simulink model "mdl4"  (Simulink 8.3)
settings: Solver=FixedStepDiscrete  SolverMode=SingleTasking  StartTime=TIME(1)  StopTime=TIME(end)  FixedStep=SIMSTEP  RelTol=1e-3
values from neighbouring files (symbols this model uses):
  Parameter113 = 123    [scr_simdata_all.mat]
  Parameter131 = 3    [scr_simdata_all.mat]
  Parameter132 = 100    [scr_simdata_all.mat]
  Parameter144 = 3    [scr_simdata_all.mat]
  Parameter51 = 0    [scr_simdata_all.mat]
  Parameter52 = 1    [scr_simdata_all.mat]
  Parameter53 = 2    [scr_simdata_all.mat]
  Parameter54 = 255    [scr_simdata_all.mat]
  Parameter69 = 27    [scr_simdata_all.mat]
  Parameter91 = 75    [scr_simdata_all.mat]
  SIMSTEP = 0.0001024    [scr_simdata_all.mat]
(part 2 of 4)

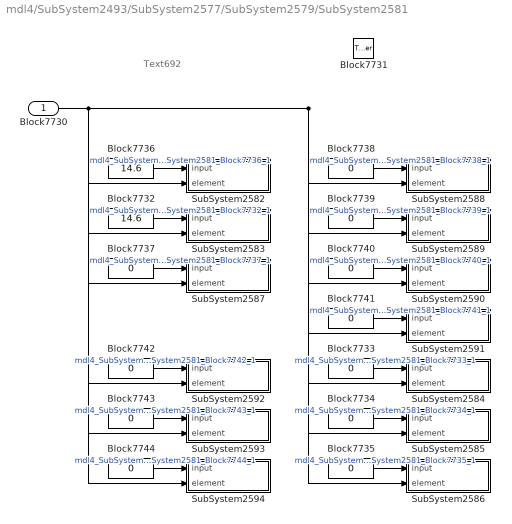
== system mdl4/SubSystem2493/SubSystem2577/SubSystem2579/SubSystem2581 ==
  note: Text692
  Block7730 : Inport
  Block7731 : TriggerPort  TriggerType=function-call
  Block7732 : Constant  Value=14.6  OutDataTypeStr=double  SampleTime=-1
  Block{7733..7735,7737..7744} (11 alike) : Constant  Value=0  OutDataTypeStr=double  SampleTime=-1
  Block7736 : Constant  Value=14.6  OutDataTypeStr=double  SampleTime=-1
  SubSystem2582 : Subsystem  TreatAsAtomicUnit=on  mask(***ATC.DSWVEC***){bd_version=1.01.A, r0=DSM258, r1=-1, r2=, r3=, r4=, r5=, r6=, r7=, r8=, r9=, c0=, c1=, c2=, c3=, c4=, c5=, c6=, c7=, c8=, c9=}
      mask prompts: bd_version "Version"
      mask help: これはAutoCからのブロックです．編集禁止．
      settings: OpenFcn=warndlg('変更禁止!');
      mask Help: web(ui_blockhelpmng(gcb));
      mask Display: disp('ATC.DSRVEC')
  SubSystem2583 : Subsystem  TreatAsAtomicUnit=on  mask(***ATC.DSWVEC***){bd_version=1.01.A, r0=DSM275, r1=-1, r2=, r3=, r4=, r5=, r6=, r7=, r8=, r9=, c0=, c1=, c2=, c3=, c4=, c5=, c6=, c7=, c8=, c9=}
      mask prompts: bd_version "Version"
      mask help: これはAutoCからのブロックです．編集禁止．
      settings: OpenFcn=warndlg('変更禁止!');
      mask Help: web(ui_blockhelpmng(gcb));
      mask Display: disp('ATC.DSRVEC')
  SubSystem2584 : Subsystem  TreatAsAtomicUnit=on  mask(***ATC.DSWVEC***){bd_version=1.01.A, r0=DSM295, r1=-1, r2=, r3=, r4=, r5=, r6=, r7=, r8=, r9=, c0=, c1=, c2=, c3=, c4=, c5=, c6=, c7=, c8=, c9=}
      mask prompts: bd_version "Version"
      mask help: これはAutoCからのブロックです．編集禁止．
      settings: OpenFcn=warndlg('変更禁止!');
      mask Help: web(ui_blockhelpmng(gcb));
      mask Display: disp('ATC.DSRVEC')
  SubSystem2585 : Subsystem  TreatAsAtomicUnit=on  mask(***ATC.DSWVEC***){bd_version=1.01.A, r0=DSM280, r1=-1, r2=, r3=, r4=, r5=, r6=, r7=, r8=, r9=, c0=, c1=, c2=, c3=, c4=, c5=, c6=, c7=, c8=, c9=}
      mask prompts: bd_version "Version"
      mask help: これはAutoCからのブロックです．編集禁止．
      settings: OpenFcn=warndlg('変更禁止!');
      mask Help: web(ui_blockhelpmng(gcb));
      mask Display: disp('ATC.DSRVEC')
  SubSystem2586 : Subsystem  TreatAsAtomicUnit=on  mask(***ATC.DSWVEC***){bd_version=1.01.A, r0=DSM282, r1=-1, r2=, r3=, r4=, r5=, r6=, r7=, r8=, r9=, c0=, c1=, c2=, c3=, c4=, c5=, c6=, c7=, c8=, c9=}
      mask prompts: bd_version "Version"
      mask help: これはAutoCからのブロックです．編集禁止．
      settings: OpenFcn=warndlg('変更禁止!');
      mask Help: web(ui_blockhelpmng(gcb));
      mask Display: disp('ATC.DSRVEC')
  SubSystem2587 : Subsystem  TreatAsAtomicUnit=on  mask(***ATC.DSWVEC***){bd_version=1.01.A, r0=DSM274, r1=-1, r2=, r3=, r4=, r5=, r6=, r7=, r8=, r9=, c0=, c1=, c2=, c3=, c4=, c5=, c6=, c7=, c8=, c9=}
      mask prompts: bd_version "Version"
      mask help: これはAutoCからのブロックです．編集禁止．
      settings: OpenFcn=warndlg('変更禁止!');
      mask Help: web(ui_blockhelpmng(gcb));
      mask Display: disp('ATC.DSRVEC')
  SubSystem2588 : Subsystem  TreatAsAtomicUnit=on  mask(***ATC.DSWVEC***){bd_version=1.01.A, r0=DSM302, r1=-1, r2=, r3=, r4=, r5=, r6=, r7=, r8=, r9=, c0=, c1=, c2=, c3=, c4=, c5=, c6=, c7=, c8=, c9=}
      mask prompts: bd_version "Version"
      mask help: これはAutoCからのブロックです．編集禁止．
      settings: OpenFcn=warndlg('変更禁止!');
      mask Help: web(ui_blockhelpmng(gcb));
      mask Display: disp('ATC.DSRVEC')
  SubSystem2589 : Subsystem  TreatAsAtomicUnit=on  mask(***ATC.DSWVEC***){bd_version=1.01.A, r0=DSM303, r1=-1, r2=, r3=, r4=, r5=, r6=, r7=, r8=, r9=, c0=, c1=, c2=, c3=, c4=, c5=, c6=, c7=, c8=, c9=}
      mask prompts: bd_version "Version"
      mask help: これはAutoCからのブロックです．編集禁止．
      settings: OpenFcn=warndlg('変更禁止!');
      mask Help: web(ui_blockhelpmng(gcb));
      mask Display: disp('ATC.DSRVEC')
  SubSystem2590 : Subsystem  TreatAsAtomicUnit=on  mask(***ATC.DSWVEC***){bd_version=1.01.A, r0=DSM300, r1=-1, r2=, r3=, r4=, r5=, r6=, r7=, r8=, r9=, c0=, c1=, c2=, c3=, c4=, c5=, c6=, c7=, c8=, c9=}
      mask prompts: bd_version "Version"
      mask help: これはAutoCからのブロックです．編集禁止．
      settings: OpenFcn=warndlg('変更禁止!');
      mask Help: web(ui_blockhelpmng(gcb));
      mask Display: disp('ATC.DSRVEC')
  SubSystem2591 : Subsystem  TreatAsAtomicUnit=on  mask(***ATC.DSWVEC***){bd_version=1.01.A, r0=DSM301, r1=-1, r2=, r3=, r4=, r5=, r6=, r7=, r8=, r9=, c0=, c1=, c2=, c3=, c4=, c5=, c6=, c7=, c8=, c9=}
      mask prompts: bd_version "Version"
      mask help: これはAutoCからのブロックです．編集禁止．
      settings: OpenFcn=warndlg('変更禁止!');
      mask Help: web(ui_blockhelpmng(gcb));
      mask Display: disp('ATC.DSRVEC')
  SubSystem2592 : Subsystem  TreatAsAtomicUnit=on  mask(***ATC.DSWVEC***){bd_version=1.01.A, r0=DSM293, r1=-1, r2=, r3=, r4=, r5=, r6=, r7=, r8=, r9=, c0=, c1=, c2=, c3=, c4=, c5=, c6=, c7=, c8=, c9=}
      mask prompts: bd_version "Version"
      mask help: これはAutoCからのブロックです．編集禁止．
      settings: OpenFcn=warndlg('変更禁止!');
      mask Help: web(ui_blockhelpmng(gcb));
      mask Display: disp('ATC.DSRVEC')
  SubSystem2593 : Subsystem  TreatAsAtomicUnit=on  mask(***ATC.DSWVEC***){bd_version=1.01.A, r0=DSM279, r1=-1, r2=, r3=, r4=, r5=, r6=, r7=, r8=, r9=, c0=, c1=, c2=, c3=, c4=, c5=, c6=, c7=, c8=, c9=}
      mask prompts: bd_version "Version"
      mask help: これはAutoCからのブロックです．編集禁止．
      settings: OpenFcn=warndlg('変更禁止!');
      mask Help: web(ui_blockhelpmng(gcb));
      mask Display: disp('ATC.DSRVEC')
  SubSystem2594 : Subsystem  TreatAsAtomicUnit=on  mask(***ATC.DSWVEC***){bd_version=1.01.A, r0=DSM281, r1=-1, r2=, r3=, r4=, r5=, r6=, r7=, r8=, r9=, c0=, c1=, c2=, c3=, c4=, c5=, c6=, c7=, c8=, c9=}
      mask prompts: bd_version "Version"
      mask help: これはAutoCからのブロックです．編集禁止．
      settings: OpenFcn=warndlg('変更禁止!');
      mask Help: web(ui_blockhelpmng(gcb));
      mask Display: disp('ATC.DSRVEC')
  wires:
  Block7736/1 -> SubSystem2582/1(input)  "mdl4_SubSystem2493_SubSystem2577_SubSystem2579_SubSystem2581_Block7736_1"
  Block7730/1 -> SubSystem2582/2(element), SubSystem2587/2(element), SubSystem2583/2(element), SubSystem2592/2(element), SubSystem2593/2(element), SubSystem2594/2(element), SubSystem2588/2(element), SubSystem2589/2(element), SubSystem2590/2(element), SubSystem2591/2(element), SubSystem2584/2(element), SubSystem2585/2(element), SubSystem2586/2(element)
  Block7732/1 -> SubSystem2583/1(input)  "mdl4_SubSystem2493_SubSystem2577_SubSystem2579_SubSystem2581_Block7732_1"
  Block7737/1 -> SubSystem2587/1(input)  "mdl4_SubSystem2493_SubSystem2577_SubSystem2579_SubSystem2581_Block7737_1"
  Block7738/1 -> SubSystem2588/1(input)  "mdl4_SubSystem2493_SubSystem2577_SubSystem2579_SubSystem2581_Block7738_1"
  Block7739/1 -> SubSystem2589/1(input)  "mdl4_SubSystem2493_SubSystem2577_SubSystem2579_SubSystem2581_Block7739_1"
  Block7740/1 -> SubSystem2590/1(input)  "mdl4_SubSystem2493_SubSystem2577_SubSystem2579_SubSystem2581_Block7740_1"
  Block7741/1 -> SubSystem2591/1(input)  "mdl4_SubSystem2493_SubSystem2577_SubSystem2579_SubSystem2581_Block7741_1"
  Block7742/1 -> SubSystem2592/1(input)  "mdl4_SubSystem2493_SubSystem2577_SubSystem2579_SubSystem2581_Block7742_1"
  Block7743/1 -> SubSystem2593/1(input)  "mdl4_SubSystem2493_SubSystem2577_SubSystem2579_SubSystem2581_Block7743_1"
  Block7744/1 -> SubSystem2594/1(input)  "mdl4_SubSystem2493_SubSystem2577_SubSystem2579_SubSystem2581_Block7744_1"
  Block7733/1 -> SubSystem2584/1(input)  "mdl4_SubSystem2493_SubSystem2577_SubSystem2579_SubSystem2581_Block7733_1"
  Block7734/1 -> SubSystem2585/1(input)  "mdl4_SubSystem2493_SubSystem2577_SubSystem2579_SubSystem2581_Block7734_1"
  Block7735/1 -> SubSystem2586/1(input)  "mdl4_SubSystem2493_SubSystem2577_SubSystem2579_SubSystem2581_Block7735_1"

== system mdl4/SubSystem2493/SubSystem2494/SubSystem2500/SubSystem2504/SubSystem2505 ==
  note: ***編集禁止***
  input : Inport
  element : Inport  Port=2
  Assignment : Assignment  IndexOptions=Index vector (port)  OutputSizes=[1 1]
  Inside_DSR : DataStoreRead  DataStoreName=DSM274
  Inside_DSW : DataStoreWrite  DataStoreName=DSM274
  wires:
  Assignment/1 -> Inside_DSW/1  "mdl4_SubSystem2493_SubSystem2494_SubSystem2500_SubSystem2504_SubSystem2505_Assignment_1"
  Inside_DSR/1 -> Assignment/1  "mdl4_SubSystem2493_SubSystem2494_SubSystem2500_SubSystem2504_SubSystem2505_Inside_DSR_1"
  input/1 -> Assignment/2
  element/1 -> Assignment/3

== system mdl4/SubSystem2493/SubSystem2494/SubSystem2500/SubSystem2504/SubSystem2506 ==
  note: ***編集禁止***
  In1 : Inport
  In2 : Inport  Port=2
  RO1 : RelationalOperator  Operator===  InputSameDT=on
  single1 : DataTypeConversion  OutDataTypeStr=single  SaturateOnIntegerOverflow=on  RndMeth=Zero
  single2 : DataTypeConversion  OutDataTypeStr=single  SaturateOnIntegerOverflow=on  RndMeth=Zero
  Out1 : Outport
  wires:
  single2/1 -> RO1/2  "mdl4_SubSystem2493_SubSystem2494_SubSystem2500_SubSystem2504_SubSystem2506_single2_1"
  single1/1 -> RO1/1  "mdl4_SubSystem2493_SubSystem2494_SubSystem2500_SubSystem2504_SubSystem2506_single1_1"
  In1/1 -> single1/1
  In2/1 -> single2/1
  RO1/1 -> Out1/1  "mdl4_SubSystem2493_SubSystem2494_SubSystem2500_SubSystem2504_SubSystem2506_RO1_1"

== system mdl4/SubSystem2493/SubSystem2494/SubSystem2500/SubSystem2504/SubSystem2507 ==
  note: Text615
  note: Text614
  note: Text613
  note: Text612
  Block7508 : Inport
  Block7509 : Constant  OutDataTypeStr=double  SampleTime=-1
  Block7510 : DataStoreRead  DataStoreName=DSM299
  Block7511 : DataStoreRead  DataStoreName=DSM297
  Block7512 : DataStoreRead  DataStoreName=DSM285
  Block7513 : DataStoreRead  DataStoreName=DSM283
  Block7514 : Demux  Outputs=2
  Block7517 : Sum  Inputs=+-|  OutDataTypeStr=double  RndMeth=Zero  SaturateOnIntegerOverflow=on  InputSameDT=on
  Block7518 : Switch  Threshold=0.5  RndMeth=Zero  SaturateOnIntegerOverflow=on  InputSameDT=on
  SubSystem2508 : Subsystem
  Block7519 : Outport
  Block7520 : Outport  Port=2
  Block7521 : Outport  Port=3
  Block7522 : Outport  Port=4
  wires:
  Block7510/1 -> SubSystem2508/1(In1)  "mdl4_SubSystem2493_SubSystem2494_SubSystem2500_SubSystem2504_SubSystem2507_Block7510_1"
  Block7509/1 -> SubSystem2508/2(In2)  "mdl4_SubSystem2493_SubSystem2494_SubSystem2500_SubSystem2504_SubSystem2507_Block7509_1"
  SubSystem2508/1(Out1) -> Block7518/2
  Block7508/1 -> Block7517/2
  Block7511/1 -> Block7517/1  "mdl4_SubSystem2493_SubSystem2494_SubSystem2500_SubSystem2504_SubSystem2507_Block7511_1"
  Block7517/1 -> Block7514/1  "mdl4_SubSystem2493_SubSystem2494_SubSystem2500_SubSystem2504_SubSystem2507_Block7517_1"
  Block7518/1 -> Block7519/1  "mdl4_SubSystem2493_SubSystem2494_SubSystem2500_SubSystem2504_SubSystem2507_Block7518_1"
  Block7514/1 -> Block7518/3, Block7520/1  "SigLabel273"
  Block7514/2 -> [TagName60]  "SigLabel270"
  [TagName60] -> Block7518/1  "SigLabel269"
  Block7512/1 -> Block7521/1  "mdl4_SubSystem2493_SubSystem2494_SubSystem2500_SubSystem2504_SubSystem2507_Block7512_1"
  Block7513/1 -> Block7522/1  "mdl4_SubSystem2493_SubSystem2494_SubSystem2500_SubSystem2504_SubSystem2507_Block7513_1"

== system mdl4/SubSystem2493/SubSystem2494/SubSystem2500/SubSystem2504/SubSystem2509 ==
  note: Text619
  note: Text618
  note: Text617
  note: Text616
  Block7523 : Inport
  Block7524 : Constant  OutDataTypeStr=double  SampleTime=-1
  Block7525 : DataStoreRead  DataStoreName=DSM299
  Block7526 : DataStoreRead  DataStoreName=DSM298
  Block7527 : DataStoreRead  DataStoreName=DSM286
  Block7528 : DataStoreRead  DataStoreName=DSM284
  Block7529 : Demux  Outputs=2
  Block7530 : Sum  Inputs=+-|  OutDataTypeStr=double  RndMeth=Zero  SaturateOnIntegerOverflow=on  InputSameDT=on
  Block7531 : Switch  Threshold=0.5  RndMeth=Zero  SaturateOnIntegerOverflow=on  InputSameDT=on
  SubSystem2510 : Subsystem
  Block7532 : Outport
  Block7533 : Outport  Port=2
  Block7534 : Outport  Port=3
  Block7535 : Outport  Port=4
  wires:
  Block7528/1 -> Block7535/1  "mdl4_SubSystem2493_SubSystem2494_SubSystem2500_SubSystem2504_SubSystem2509_Block7528_1"
  Block7527/1 -> Block7534/1  "mdl4_SubSystem2493_SubSystem2494_SubSystem2500_SubSystem2504_SubSystem2509_Block7527_1"
  Block7529/1 -> Block7533/1, Block7531/1  "SigLabel277"
  Block7531/1 -> Block7532/1  "mdl4_SubSystem2493_SubSystem2494_SubSystem2500_SubSystem2504_SubSystem2509_Block7531_1"
  Block7530/1 -> Block7529/1  "mdl4_SubSystem2493_SubSystem2494_SubSystem2500_SubSystem2504_SubSystem2509_Block7530_1"
  Block7526/1 -> Block7530/1  "mdl4_SubSystem2493_SubSystem2494_SubSystem2500_SubSystem2504_SubSystem2509_Block7526_1"
  Block7523/1 -> Block7530/2
  SubSystem2510/1(Out1) -> Block7531/2
  Block7524/1 -> SubSystem2510/2(In2)  "mdl4_SubSystem2493_SubSystem2494_SubSystem2500_SubSystem2504_SubSystem2509_Block7524_1"
  Block7525/1 -> SubSystem2510/1(In1)  "mdl4_SubSystem2493_SubSystem2494_SubSystem2500_SubSystem2504_SubSystem2509_Block7525_1"
  Block7529/2 -> Block7531/3  "SigLabel274"

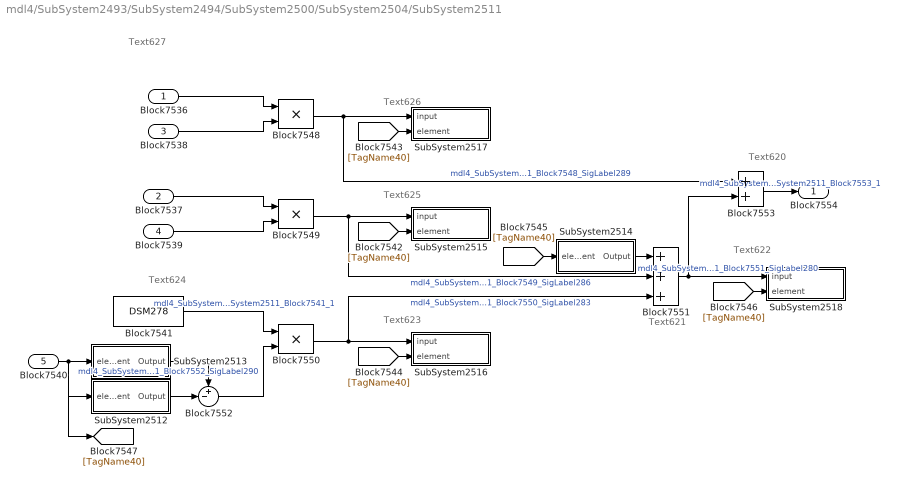
== system mdl4/SubSystem2493/SubSystem2494/SubSystem2500/SubSystem2504/SubSystem2511 ==
  note: Text627
  note: Text626
  note: Text625
  note: Text624
  note: Text623
  note: Text622
  note: Text621
  note: Text620
  Block7536 : Inport
  Block7537 : Inport  Port=2
  Block7538 : Inport  Port=3
  Block7539 : Inport  Port=4
  Block7540 : Inport  Port=5
  Block7541 : DataStoreRead  DataStoreName=DSM278
  Block7548 : Product  OutDataTypeStr=double  SaturateOnIntegerOverflow=on  RndMeth=Zero  InputSameDT=on
  Block7549 : Product  OutDataTypeStr=double  SaturateOnIntegerOverflow=on  RndMeth=Zero  InputSameDT=on
  Block7550 : Product  OutDataTypeStr=double  SaturateOnIntegerOverflow=on  RndMeth=Zero  InputSameDT=on
  Block7551 : Sum  Inputs=3  OutDataTypeStr=double  RndMeth=Zero  SaturateOnIntegerOverflow=on  InputSameDT=on
  Block7552 : Sum  Inputs=+-|  OutDataTypeStr=double  RndMeth=Zero  SaturateOnIntegerOverflow=on  InputSameDT=on
  Block7553 : Sum  Inputs=2  OutDataTypeStr=double  RndMeth=Zero  SaturateOnIntegerOverflow=on  InputSameDT=on
  SubSystem2512 : Subsystem  TreatAsAtomicUnit=on  mask(***ATC.DSRVEC***){bd_version=1.01.A, r0=DSM258, r1=-1, r2=, r3=, r4=, r5=, r6=, r7=, r8=, r9=, c0=, c1=, c2=, c3=, c4=, c5=, c6=, c7=, c8=, c9=}
      mask prompts: bd_version "Version"
      mask help: これはAutoCからのブロックです．編集禁止．
      settings: OpenFcn=warndlg('変更禁止!');
      mask Help: web(ui_blockhelpmng(gcb));
      mask Display: disp('ATC.DSRVEC')
  SubSystem2513 : Subsystem  TreatAsAtomicUnit=on  mask(***ATC.DSRVEC***){bd_version=1.01.A, r0=DSM259, r1=-1, r2=, r3=, r4=, r5=, r6=, r7=, r8=, r9=, c0=, c1=, c2=, c3=, c4=, c5=, c6=, c7=, c8=, c9=}
      mask prompts: bd_version "Version"
      mask help: これはAutoCからのブロックです．編集禁止．
      settings: OpenFcn=warndlg('変更禁止!');
      mask Help: web(ui_blockhelpmng(gcb));
      mask Display: disp('ATC.DSRVEC')
  SubSystem2514 : Subsystem  TreatAsAtomicUnit=on  mask(***ATC.DSRVEC***){bd_version=1.01.A, r0=DSM300, r1=-1, r2=, r3=, r4=, r5=, r6=, r7=, r8=, r9=, c0=, c1=, c2=, c3=, c4=, c5=, c6=, c7=, c8=, c9=}
      mask prompts: bd_version "Version"
      mask help: これはAutoCからのブロックです．編集禁止．
      settings: OpenFcn=warndlg('変更禁止!');
      mask Help: web(ui_blockhelpmng(gcb));
      mask Display: disp('ATC.DSRVEC')
  SubSystem2515 : Subsystem  TreatAsAtomicUnit=on  mask(***ATC.DSWVEC***){bd_version=1.01.A, r0=DSM302, r1=-1, r2=, r3=, r4=, r5=, r6=, r7=, r8=, r9=, c0=, c1=, c2=, c3=, c4=, c5=, c6=, c7=, c8=, c9=}
      mask prompts: bd_version "Version"
      mask help: これはAutoCからのブロックです．編集禁止．
      settings: OpenFcn=warndlg('変更禁止!');
      mask Help: web(ui_blockhelpmng(gcb));
      mask Display: disp('ATC.DSRVEC')
  SubSystem2516 : Subsystem  TreatAsAtomicUnit=on  mask(***ATC.DSWVEC***){bd_version=1.01.A, r0=DSM301, r1=-1, r2=, r3=, r4=, r5=, r6=, r7=, r8=, r9=, c0=, c1=, c2=, c3=, c4=, c5=, c6=, c7=, c8=, c9=}
      mask prompts: bd_version "Version"
      mask help: これはAutoCからのブロックです．編集禁止．
      settings: OpenFcn=warndlg('変更禁止!');
      mask Help: web(ui_blockhelpmng(gcb));
      mask Display: disp('ATC.DSRVEC')
  SubSystem2517 : Subsystem  TreatAsAtomicUnit=on  mask(***ATC.DSWVEC***){bd_version=1.01.A, r0=DSM303, r1=-1, r2=, r3=, r4=, r5=, r6=, r7=, r8=, r9=, c0=, c1=, c2=, c3=, c4=, c5=, c6=, c7=, c8=, c9=}
      mask prompts: bd_version "Version"
      mask help: これはAutoCからのブロックです．編集禁止．
      settings: OpenFcn=warndlg('変更禁止!');
      mask Help: web(ui_blockhelpmng(gcb));
      mask Display: disp('ATC.DSRVEC')
  SubSystem2518 : Subsystem  TreatAsAtomicUnit=on  mask(***ATC.DSWVEC***){bd_version=1.01.A, r0=DSM300, r1=-1, r2=, r3=, r4=, r5=, r6=, r7=, r8=, r9=, c0=, c1=, c2=, c3=, c4=, c5=, c6=, c7=, c8=, c9=}
      mask prompts: bd_version "Version"
      mask help: これはAutoCからのブロックです．編集禁止．
      settings: OpenFcn=warndlg('変更禁止!');
      mask Help: web(ui_blockhelpmng(gcb));
      mask Display: disp('ATC.DSRVEC')
  Block7554 : Outport
  wires:
  SubSystem2512/1(Output) -> Block7552/2
  SubSystem2513/1(Output) -> Block7552/1
  Block7540/1 -> SubSystem2513/1(element), SubSystem2512/1(element), [TagName40]
  Block7552/1 -> Block7550/2  "mdl4_SubSystem2493_SubSystem2494_SubSystem2500_SubSystem2504_SubSystem2511_Block7552_SigLabel290"
  Block7548/1 -> SubSystem2517/1(input), Block7553/1  "mdl4_SubSystem2493_SubSystem2494_SubSystem2500_SubSystem2504_SubSystem2511_Block7548_SigLabel289"
  [TagName40] -> SubSystem2517/2(element)
  Block7549/1 -> SubSystem2515/1(input), Block7551/2  "mdl4_SubSystem2493_SubSystem2494_SubSystem2500_SubSystem2504_SubSystem2511_Block7549_SigLabel286"
  [TagName40] -> SubSystem2515/2(element)
  Block7541/1 -> Block7550/1  "mdl4_SubSystem2493_SubSystem2494_SubSystem2500_SubSystem2504_SubSystem2511_Block7541_1"
  Block7550/1 -> SubSystem2516/1(input), Block7551/3  "mdl4_SubSystem2493_SubSystem2494_SubSystem2500_SubSystem2504_SubSystem2511_Block7550_SigLabel283"
  [TagName40] -> SubSystem2516/2(element)
  [TagName40] -> SubSystem2514/1(element)
  [TagName40] -> SubSystem2518/2(element)
  SubSystem2514/1(Output) -> Block7551/1
  Block7551/1 -> SubSystem2518/1(input), Block7553/2  "mdl4_SubSystem2493_SubSystem2494_SubSystem2500_SubSystem2504_SubSystem2511_Block7551_SigLabel280"
  Block7553/1 -> Block7554/1  "mdl4_SubSystem2493_SubSystem2494_SubSystem2500_SubSystem2504_SubSystem2511_Block7553_1"
  Block7536/1 -> Block7548/1
  Block7538/1 -> Block7548/2
  Block7537/1 -> Block7549/1
  Block7539/1 -> Block7549/2

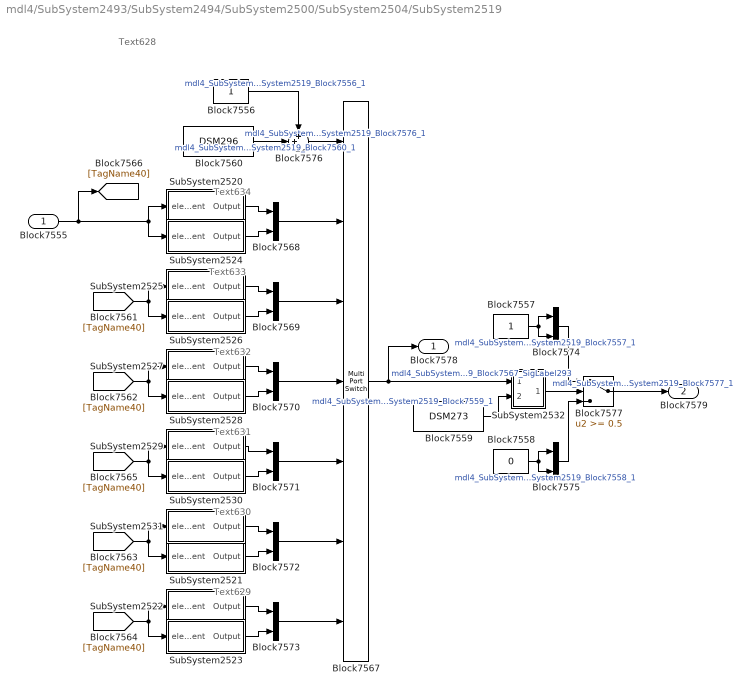
== system mdl4/SubSystem2493/SubSystem2494/SubSystem2500/SubSystem2504/SubSystem2519 ==
  note: Text634
  note: Text633
  note: Text632
  note: Text631
  note: Text630
  note: Text629
  note: Text628
  Block7555 : Inport
  Block7556 : Constant  OutDataTypeStr=double  SampleTime=-1
  Block7557 : Constant  OutDataTypeStr=double  SampleTime=-1
  Block7558 : Constant  Value=0  OutDataTypeStr=double  SampleTime=-1
  Block7559 : DataStoreRead  DataStoreName=DSM273
  Block7560 : DataStoreRead  DataStoreName=DSM296
  Block7567 : MultiPortSwitch  Inputs=6  RndMeth=Zero  SaturateOnIntegerOverflow=on  InputSameDT=on
  Block{7568..7575} (8 alike) : Mux  Inputs=2
  Block7576 : Sum  Inputs=++|  OutDataTypeStr=double  RndMeth=Zero  SaturateOnIntegerOverflow=on  InputSameDT=on
  Block7577 : Switch  Threshold=0.5  RndMeth=Zero  SaturateOnIntegerOverflow=on  InputSameDT=on
  SubSystem2520 : Subsystem  TreatAsAtomicUnit=on  mask(***ATC.DSRVEC***){bd_version=1.01.A, r0=DSM114, r1=-1, r2=, r3=, r4=, r5=, r6=, r7=, r8=, r9=, c0=, c1=, c2=, c3=, c4=, c5=, c6=, c7=, c8=, c9=}
      mask prompts: bd_version "Version"
      mask help: これはAutoCからのブロックです．編集禁止．
      settings: OpenFcn=warndlg('変更禁止!');
      mask Help: web(ui_blockhelpmng(gcb));
      mask Display: disp('ATC.DSRVEC')
  SubSystem2521 : Subsystem  TreatAsAtomicUnit=on  mask(***ATC.DSRVEC***){bd_version=1.01.A, r0=DSM105, r1=-1, r2=, r3=, r4=, r5=, r6=, r7=, r8=, r9=, c0=, c1=, c2=, c3=, c4=, c5=, c6=, c7=, c8=, c9=}
      mask prompts: bd_version "Version"
      mask help: これはAutoCからのブロックです．編集禁止．
      settings: OpenFcn=warndlg('変更禁止!');
      mask Help: web(ui_blockhelpmng(gcb));
      mask Display: disp('ATC.DSRVEC')
  SubSystem2522 : Subsystem  TreatAsAtomicUnit=on  mask(***ATC.DSRVEC***){bd_version=1.01.A, r0=DSM111, r1=-1, r2=, r3=, r4=, r5=, r6=, r7=, r8=, r9=, c0=, c1=, c2=, c3=, c4=, c5=, c6=, c7=, c8=, c9=}
      mask prompts: bd_version "Version"
      mask help: これはAutoCからのブロックです．編集禁止．
      settings: OpenFcn=warndlg('変更禁止!');
      mask Help: web(ui_blockhelpmng(gcb));
      mask Display: disp('ATC.DSRVEC')
  SubSystem2523 : Subsystem  TreatAsAtomicUnit=on  mask(***ATC.DSRVEC***){bd_version=1.01.A, r0=DSM113, r1=-1, r2=, r3=, r4=, r5=, r6=, r7=, r8=, r9=, c0=, c1=, c2=, c3=, c4=, c5=, c6=, c7=, c8=, c9=}
      mask prompts: bd_version "Version"
      mask help: これはAutoCからのブロックです．編集禁止．
      settings: OpenFcn=warndlg('変更禁止!');
      mask Help: web(ui_blockhelpmng(gcb));
      mask Display: disp('ATC.DSRVEC')
  SubSystem2524 : Subsystem  TreatAsAtomicUnit=on  mask(***ATC.DSRVEC***){bd_version=1.01.A, r0=DSM118, r1=-1, r2=, r3=, r4=, r5=, r6=, r7=, r8=, r9=, c0=, c1=, c2=, c3=, c4=, c5=, c6=, c7=, c8=, c9=}
      mask prompts: bd_version "Version"
      mask help: これはAutoCからのブロックです．編集禁止．
      settings: OpenFcn=warndlg('変更禁止!');
      mask Help: web(ui_blockhelpmng(gcb));
      mask Display: disp('ATC.DSRVEC')
  SubSystem2525 : Subsystem  TreatAsAtomicUnit=on  mask(***ATC.DSRVEC***){bd_version=1.01.A, r0=DSM117, r1=-1, r2=, r3=, r4=, r5=, r6=, r7=, r8=, r9=, c0=, c1=, c2=, c3=, c4=, c5=, c6=, c7=, c8=, c9=}
      mask prompts: bd_version "Version"
      mask help: これはAutoCからのブロックです．編集禁止．
      settings: OpenFcn=warndlg('変更禁止!');
      mask Help: web(ui_blockhelpmng(gcb));
      mask Display: disp('ATC.DSRVEC')
  SubSystem2526 : Subsystem  TreatAsAtomicUnit=on  mask(***ATC.DSRVEC***){bd_version=1.01.A, r0=DSM121, r1=-1, r2=, r3=, r4=, r5=, r6=, r7=, r8=, r9=, c0=, c1=, c2=, c3=, c4=, c5=, c6=, c7=, c8=, c9=}
      mask prompts: bd_version "Version"
      mask help: これはAutoCからのブロックです．編集禁止．
      settings: OpenFcn=warndlg('変更禁止!');
      mask Help: web(ui_blockhelpmng(gcb));
      mask Display: disp('ATC.DSRVEC')
  SubSystem2527 : Subsystem  TreatAsAtomicUnit=on  mask(***ATC.DSRVEC***){bd_version=1.01.A, r0=DSM124, r1=-1, r2=, r3=, r4=, r5=, r6=, r7=, r8=, r9=, c0=, c1=, c2=, c3=, c4=, c5=, c6=, c7=, c8=, c9=}
      mask prompts: bd_version "Version"
      mask help: これはAutoCからのブロックです．編集禁止．
      settings: OpenFcn=warndlg('変更禁止!');
      mask Help: web(ui_blockhelpmng(gcb));
      mask Display: disp('ATC.DSRVEC')
  SubSystem2528 : Subsystem  TreatAsAtomicUnit=on  mask(***ATC.DSRVEC***){bd_version=1.01.A, r0=DSM127, r1=-1, r2=, r3=, r4=, r5=, r6=, r7=, r8=, r9=, c0=, c1=, c2=, c3=, c4=, c5=, c6=, c7=, c8=, c9=}
      mask prompts: bd_version "Version"
      mask help: これはAutoCからのブロックです．編集禁止．
      settings: OpenFcn=warndlg('変更禁止!');
      mask Help: web(ui_blockhelpmng(gcb));
      mask Display: disp('ATC.DSRVEC')
  SubSystem2529 : Subsystem  TreatAsAtomicUnit=on  mask(***ATC.DSRVEC***){bd_version=1.01.A, r0=DSM107, r1=-1, r2=, r3=, r4=, r5=, r6=, r7=, r8=, r9=, c0=, c1=, c2=, c3=, c4=, c5=, c6=, c7=, c8=, c9=}
      mask prompts: bd_version "Version"
      mask help: これはAutoCからのブロックです．編集禁止．
      settings: OpenFcn=warndlg('変更禁止!');
      mask Help: web(ui_blockhelpmng(gcb));
      mask Display: disp('ATC.DSRVEC')
  SubSystem2530 : Subsystem  TreatAsAtomicUnit=on  mask(***ATC.DSRVEC***){bd_version=1.01.A, r0=DSM109, r1=-1, r2=, r3=, r4=, r5=, r6=, r7=, r8=, r9=, c0=, c1=, c2=, c3=, c4=, c5=, c6=, c7=, c8=, c9=}
      mask prompts: bd_version "Version"
      mask help: これはAutoCからのブロックです．編集禁止．
      settings: OpenFcn=warndlg('変更禁止!');
      mask Help: web(ui_blockhelpmng(gcb));
      mask Display: disp('ATC.DSRVEC')
  SubSystem2531 : Subsystem  TreatAsAtomicUnit=on  mask(***ATC.DSRVEC***){bd_version=1.01.A, r0=DSM103, r1=-1, r2=, r3=, r4=, r5=, r6=, r7=, r8=, r9=, c0=, c1=, c2=, c3=, c4=, c5=, c6=, c7=, c8=, c9=}
      mask prompts: bd_version "Version"
      mask help: これはAutoCからのブロックです．編集禁止．
      settings: OpenFcn=warndlg('変更禁止!');
      mask Help: web(ui_blockhelpmng(gcb));
      mask Display: disp('ATC.DSRVEC')
  SubSystem2532 : Subsystem
  Block7578 : Outport
  Block7579 : Outport  Port=2
  wires:
  Block7560/1 -> Block7576/2  "mdl4_SubSystem2493_SubSystem2494_SubSystem2500_SubSystem2504_SubSystem2519_Block7560_1"
  Block7556/1 -> Block7576/1  "mdl4_SubSystem2493_SubSystem2494_SubSystem2500_SubSystem2504_SubSystem2519_Block7556_1"
  Block7576/1 -> Block7567/1  "mdl4_SubSystem2493_SubSystem2494_SubSystem2500_SubSystem2504_SubSystem2519_Block7576_1"
  Block7555/1 -> SubSystem2524/1(element), SubSystem2520/1(element), [TagName40]
  SubSystem2520/1(Output) -> Block7568/1
  SubSystem2524/1(Output) -> Block7568/2
  Block7568/1 -> Block7567/2
  [TagName40] -> SubSystem2525/1(element), SubSystem2526/1(element)
  SubSystem2525/1(Output) -> Block7569/1
  SubSystem2526/1(Output) -> Block7569/2
  [TagName40] -> SubSystem2527/1(element), SubSystem2528/1(element)
  SubSystem2527/1(Output) -> Block7570/1
  SubSystem2528/1(Output) -> Block7570/2
  [TagName40] -> SubSystem2529/1(element), SubSystem2530/1(element)
  SubSystem2530/1(Output) -> Block7571/2
  [TagName40] -> SubSystem2531/1(element), SubSystem2521/1(element)
  SubSystem2531/1(Output) -> Block7572/1
  SubSystem2521/1(Output) -> Block7572/2
  [TagName40] -> SubSystem2522/1(element), SubSystem2523/1(element)
  SubSystem2522/1(Output) -> Block7573/1
  SubSystem2523/1(Output) -> Block7573/2
  SubSystem2529/1(Output) -> Block7571/1
  Block7569/1 -> Block7567/3
  Block7570/1 -> Block7567/4
  Block7571/1 -> Block7567/5
  Block7572/1 -> Block7567/6
  Block7573/1 -> Block7567/7
  Block7567/1 -> Block7578/1, SubSystem2532/1(In1)  "mdl4_SubSystem2493_SubSystem2494_SubSystem2500_SubSystem2504_SubSystem2519_Block7567_SigLabel293"
  Block7559/1 -> SubSystem2532/2(In2)  "mdl4_SubSystem2493_SubSystem2494_SubSystem2500_SubSystem2504_SubSystem2519_Block7559_1"
  SubSystem2532/1(Out1) -> Block7577/2
  Block7577/1 -> Block7579/1  "mdl4_SubSystem2493_SubSystem2494_SubSystem2500_SubSystem2504_SubSystem2519_Block7577_1"
  Block7557/1 -> Block7574/1, Block7574/2  "mdl4_SubSystem2493_SubSystem2494_SubSystem2500_SubSystem2504_SubSystem2519_Block7557_1"
  Block7558/1 -> Block7575/1, Block7575/2  "mdl4_SubSystem2493_SubSystem2494_SubSystem2500_SubSystem2504_SubSystem2519_Block7558_1"
  Block7574/1 -> Block7577/1
  Block7575/1 -> Block7577/3

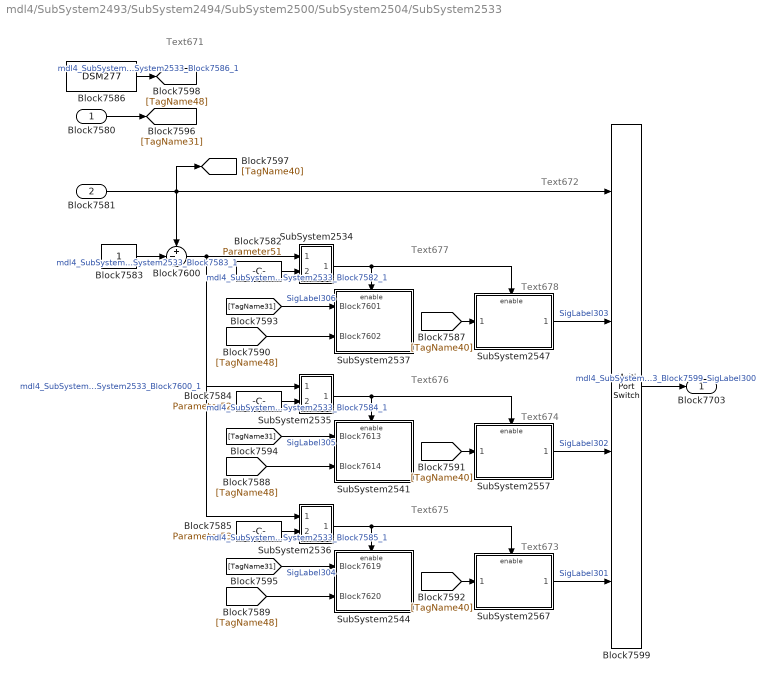
== system mdl4/SubSystem2493/SubSystem2494/SubSystem2500/SubSystem2504/SubSystem2533 ==
  note: Text678
  note: Text677
  note: Text676
  note: Text675
  note: Text674
  note: Text673
  note: Text672
  note: Text671
  Block7580 : Inport
  Block7581 : Inport  Port=2
  Block7582 : Constant  Value=Parameter51  OutDataTypeStr=double  SampleTime=-1
  Block7583 : Constant  OutDataTypeStr=double  SampleTime=-1
  Block7584 : Constant  Value=Parameter52  OutDataTypeStr=double  SampleTime=-1
  Block7585 : Constant  Value=Parameter53  OutDataTypeStr=double  SampleTime=-1
  Block7586 : DataStoreRead  DataStoreName=DSM277
  Block7599 : MultiPortSwitch  RndMeth=Zero  SaturateOnIntegerOverflow=on  InputSameDT=on
  Block7600 : Sum  Inputs=+-|  OutDataTypeStr=double  RndMeth=Zero  SaturateOnIntegerOverflow=on  InputSameDT=on
  SubSystem2534 : Subsystem
  SubSystem2535 : Subsystem
  SubSystem2536 : Subsystem
  SubSystem2537 : Subsystem  Priority=10  TreatAsAtomicUnit=on
      settings: AttributesFormatString=Attribute1933
  SubSystem2541 : Subsystem  Priority=10  TreatAsAtomicUnit=on
      settings: AttributesFormatString=Attribute1939
  SubSystem2544 : Subsystem  Priority=10  TreatAsAtomicUnit=on
      settings: AttributesFormatString=Attribute1943
  SubSystem2547 : Subsystem  Priority=20  TreatAsAtomicUnit=on
      settings: AttributesFormatString=Attribute1947
  SubSystem2557 : Subsystem  Priority=20  TreatAsAtomicUnit=on
      settings: AttributesFormatString=Attribute1954
  SubSystem2567 : Subsystem  Priority=20  TreatAsAtomicUnit=on
      settings: AttributesFormatString=Attribute1961
  Block7703 : Outport
  wires:
  Block7582/1 -> SubSystem2534/2(In2)  "mdl4_SubSystem2493_SubSystem2494_SubSystem2500_SubSystem2504_SubSystem2533_Block7582_1"
  SubSystem2534/1(Out1) -> SubSystem2537/Enable, SubSystem2547/Enable
  [TagName31] -> SubSystem2537/1(Block7601)  "SigLabel306"
  Block7584/1 -> SubSystem2535/2(In2)  "mdl4_SubSystem2493_SubSystem2494_SubSystem2500_SubSystem2504_SubSystem2533_Block7584_1"
  [TagName48] -> SubSystem2541/2(Block7614)
  SubSystem2535/1(Out1) -> SubSystem2541/Enable, SubSystem2557/Enable
  [TagName31] -> SubSystem2541/1(Block7613)  "SigLabel305"
  Block7585/1 -> SubSystem2536/2(In2)  "mdl4_SubSystem2493_SubSystem2494_SubSystem2500_SubSystem2504_SubSystem2533_Block7585_1"
  [TagName48] -> SubSystem2544/2(Block7620)
  SubSystem2536/1(Out1) -> SubSystem2544/Enable, SubSystem2567/Enable
  [TagName31] -> SubSystem2544/1(Block7619)  "SigLabel304"
  [TagName48] -> SubSystem2537/2(Block7602)
  SubSystem2547/1(Block7650) -> Block7599/2  "SigLabel303"
  SubSystem2557/1(Block7676) -> Block7599/3  "SigLabel302"
  SubSystem2567/1(Block7702) -> Block7599/4  "SigLabel301"
  Block7581/1 -> Block7599/1, Block7600/1, [TagName40]
  Block7599/1 -> Block7703/1  "mdl4_SubSystem2493_SubSystem2494_SubSystem2500_SubSystem2504_SubSystem2533_Block7599_SigLabel300"
  Block7583/1 -> Block7600/2  "mdl4_SubSystem2493_SubSystem2494_SubSystem2500_SubSystem2504_SubSystem2533_Block7583_1"
  Block7600/1 -> SubSystem2535/1(In1), SubSystem2536/1(In1), SubSystem2534/1(In1)  "mdl4_SubSystem2493_SubSystem2494_SubSystem2500_SubSystem2504_SubSystem2533_Block7600_1"
  Block7586/1 -> [TagName48]  "mdl4_SubSystem2493_SubSystem2494_SubSystem2500_SubSystem2504_SubSystem2533_Block7586_1"
  Block7580/1 -> [TagName31]
  [TagName40] -> SubSystem2547/1(Block7625)
  [TagName40] -> SubSystem2557/1(Block7651)
  [TagName40] -> SubSystem2567/1(Block7677)

== system mdl4/SubSystem2493/SubSystem2577/SubSystem2579/SubSystem2581/SubSystem2582 ==
  note: ***編集禁止***
  input : Inport
  element : Inport  Port=2
  Assignment : Assignment  IndexOptions=Index vector (port)  OutputSizes=[1 1]
  Inside_DSR : DataStoreRead  DataStoreName=DSM258
  Inside_DSW : DataStoreWrite  DataStoreName=DSM258
  wires:
  Assignment/1 -> Inside_DSW/1  "mdl4_SubSystem2493_SubSystem2577_SubSystem2579_SubSystem2581_SubSystem2582_Assignment_1"
  Inside_DSR/1 -> Assignment/1  "mdl4_SubSystem2493_SubSystem2577_SubSystem2579_SubSystem2581_SubSystem2582_Inside_DSR_1"
  input/1 -> Assignment/2
  element/1 -> Assignment/3

== system mdl4/SubSystem2493/SubSystem2577/SubSystem2579/SubSystem2581/SubSystem2583 ==
  note: ***編集禁止***
  input : Inport
  element : Inport  Port=2
  Assignment : Assignment  IndexOptions=Index vector (port)  OutputSizes=[1 1]
  Inside_DSR : DataStoreRead  DataStoreName=DSM275
  Inside_DSW : DataStoreWrite  DataStoreName=DSM275
  wires:
  Assignment/1 -> Inside_DSW/1  "mdl4_SubSystem2493_SubSystem2577_SubSystem2579_SubSystem2581_SubSystem2583_Assignment_1"
  Inside_DSR/1 -> Assignment/1  "mdl4_SubSystem2493_SubSystem2577_SubSystem2579_SubSystem2581_SubSystem2583_Inside_DSR_1"
  input/1 -> Assignment/2
  element/1 -> Assignment/3

== system mdl4/SubSystem2493/SubSystem2577/SubSystem2579/SubSystem2581/SubSystem2584 ==
  note: ***編集禁止***
  input : Inport
  element : Inport  Port=2
  Assignment : Assignment  IndexOptions=Index vector (port)  OutputSizes=[1 1]
  Inside_DSR : DataStoreRead  DataStoreName=DSM295
  Inside_DSW : DataStoreWrite  DataStoreName=DSM295
  wires:
  Assignment/1 -> Inside_DSW/1  "mdl4_SubSystem2493_SubSystem2577_SubSystem2579_SubSystem2581_SubSystem2584_Assignment_1"
  Inside_DSR/1 -> Assignment/1  "mdl4_SubSystem2493_SubSystem2577_SubSystem2579_SubSystem2581_SubSystem2584_Inside_DSR_1"
  input/1 -> Assignment/2
  element/1 -> Assignment/3

== system mdl4/SubSystem2493/SubSystem2577/SubSystem2579/SubSystem2581/SubSystem2585 ==
  note: ***編集禁止***
  input : Inport
  element : Inport  Port=2
  Assignment : Assignment  IndexOptions=Index vector (port)  OutputSizes=[1 1]
  Inside_DSR : DataStoreRead  DataStoreName=DSM280
  Inside_DSW : DataStoreWrite  DataStoreName=DSM280
  wires:
  Assignment/1 -> Inside_DSW/1  "mdl4_SubSystem2493_SubSystem2577_SubSystem2579_SubSystem2581_SubSystem2585_Assignment_1"
  Inside_DSR/1 -> Assignment/1  "mdl4_SubSystem2493_SubSystem2577_SubSystem2579_SubSystem2581_SubSystem2585_Inside_DSR_1"
  input/1 -> Assignment/2
  element/1 -> Assignment/3

== system mdl4/SubSystem2493/SubSystem2577/SubSystem2579/SubSystem2581/SubSystem2586 ==
  note: ***編集禁止***
  input : Inport
  element : Inport  Port=2
  Assignment : Assignment  IndexOptions=Index vector (port)  OutputSizes=[1 1]
  Inside_DSR : DataStoreRead  DataStoreName=DSM282
  Inside_DSW : DataStoreWrite  DataStoreName=DSM282
  wires:
  Assignment/1 -> Inside_DSW/1  "mdl4_SubSystem2493_SubSystem2577_SubSystem2579_SubSystem2581_SubSystem2586_Assignment_1"
  Inside_DSR/1 -> Assignment/1  "mdl4_SubSystem2493_SubSystem2577_SubSystem2579_SubSystem2581_SubSystem2586_Inside_DSR_1"
  input/1 -> Assignment/2
  element/1 -> Assignment/3

== system mdl4/SubSystem2493/SubSystem2577/SubSystem2579/SubSystem2581/SubSystem2587 ==
  note: ***編集禁止***
  input : Inport
  element : Inport  Port=2
  Assignment : Assignment  IndexOptions=Index vector (port)  OutputSizes=[1 1]
  Inside_DSR : DataStoreRead  DataStoreName=DSM274
  Inside_DSW : DataStoreWrite  DataStoreName=DSM274
  wires:
  Assignment/1 -> Inside_DSW/1  "mdl4_SubSystem2493_SubSystem2577_SubSystem2579_SubSystem2581_SubSystem2587_Assignment_1"
  Inside_DSR/1 -> Assignment/1  "mdl4_SubSystem2493_SubSystem2577_SubSystem2579_SubSystem2581_SubSystem2587_Inside_DSR_1"
  input/1 -> Assignment/2
  element/1 -> Assignment/3

== system mdl4/SubSystem2493/SubSystem2577/SubSystem2579/SubSystem2581/SubSystem2588 ==
  note: ***編集禁止***
  input : Inport
  element : Inport  Port=2
  Assignment : Assignment  IndexOptions=Index vector (port)  OutputSizes=[1 1]
  Inside_DSR : DataStoreRead  DataStoreName=DSM302
  Inside_DSW : DataStoreWrite  DataStoreName=DSM302
  wires:
  Assignment/1 -> Inside_DSW/1  "mdl4_SubSystem2493_SubSystem2577_SubSystem2579_SubSystem2581_SubSystem2588_Assignment_1"
  Inside_DSR/1 -> Assignment/1  "mdl4_SubSystem2493_SubSystem2577_SubSystem2579_SubSystem2581_SubSystem2588_Inside_DSR_1"
  input/1 -> Assignment/2
  element/1 -> Assignment/3

== system mdl4/SubSystem2493/SubSystem2577/SubSystem2579/SubSystem2581/SubSystem2589 ==
  note: ***編集禁止***
  input : Inport
  element : Inport  Port=2
  Assignment : Assignment  IndexOptions=Index vector (port)  OutputSizes=[1 1]
  Inside_DSR : DataStoreRead  DataStoreName=DSM303
  Inside_DSW : DataStoreWrite  DataStoreName=DSM303
  wires:
  Assignment/1 -> Inside_DSW/1  "mdl4_SubSystem2493_SubSystem2577_SubSystem2579_SubSystem2581_SubSystem2589_Assignment_1"
  Inside_DSR/1 -> Assignment/1  "mdl4_SubSystem2493_SubSystem2577_SubSystem2579_SubSystem2581_SubSystem2589_Inside_DSR_1"
  input/1 -> Assignment/2
  element/1 -> Assignment/3

== system mdl4/SubSystem2493/SubSystem2577/SubSystem2579/SubSystem2581/SubSystem2590 ==
  note: ***編集禁止***
  input : Inport
  element : Inport  Port=2
  Assignment : Assignment  IndexOptions=Index vector (port)  OutputSizes=[1 1]
  Inside_DSR : DataStoreRead  DataStoreName=DSM300
  Inside_DSW : DataStoreWrite  DataStoreName=DSM300
  wires:
  Assignment/1 -> Inside_DSW/1  "mdl4_SubSystem2493_SubSystem2577_SubSystem2579_SubSystem2581_SubSystem2590_Assignment_1"
  Inside_DSR/1 -> Assignment/1  "mdl4_SubSystem2493_SubSystem2577_SubSystem2579_SubSystem2581_SubSystem2590_Inside_DSR_1"
  input/1 -> Assignment/2
  element/1 -> Assignment/3

== system mdl4/SubSystem2493/SubSystem2577/SubSystem2579/SubSystem2581/SubSystem2591 ==
  note: ***編集禁止***
  input : Inport
  element : Inport  Port=2
  Assignment : Assignment  IndexOptions=Index vector (port)  OutputSizes=[1 1]
  Inside_DSR : DataStoreRead  DataStoreName=DSM301
  Inside_DSW : DataStoreWrite  DataStoreName=DSM301
  wires:
  Assignment/1 -> Inside_DSW/1  "mdl4_SubSystem2493_SubSystem2577_SubSystem2579_SubSystem2581_SubSystem2591_Assignment_1"
  Inside_DSR/1 -> Assignment/1  "mdl4_SubSystem2493_SubSystem2577_SubSystem2579_SubSystem2581_SubSystem2591_Inside_DSR_1"
  input/1 -> Assignment/2
  element/1 -> Assignment/3

== system mdl4/SubSystem2493/SubSystem2577/SubSystem2579/SubSystem2581/SubSystem2592 ==
  note: ***編集禁止***
  input : Inport
  element : Inport  Port=2
  Assignment : Assignment  IndexOptions=Index vector (port)  OutputSizes=[1 1]
  Inside_DSR : DataStoreRead  DataStoreName=DSM293
  Inside_DSW : DataStoreWrite  DataStoreName=DSM293
  wires:
  Assignment/1 -> Inside_DSW/1  "mdl4_SubSystem2493_SubSystem2577_SubSystem2579_SubSystem2581_SubSystem2592_Assignment_1"
  Inside_DSR/1 -> Assignment/1  "mdl4_SubSystem2493_SubSystem2577_SubSystem2579_SubSystem2581_SubSystem2592_Inside_DSR_1"
  input/1 -> Assignment/2
  element/1 -> Assignment/3

== system mdl4/SubSystem2493/SubSystem2577/SubSystem2579/SubSystem2581/SubSystem2593 ==
  note: ***編集禁止***
  input : Inport
  element : Inport  Port=2
  Assignment : Assignment  IndexOptions=Index vector (port)  OutputSizes=[1 1]
  Inside_DSR : DataStoreRead  DataStoreName=DSM279
  Inside_DSW : DataStoreWrite  DataStoreName=DSM279
  wires:
  Assignment/1 -> Inside_DSW/1  "mdl4_SubSystem2493_SubSystem2577_SubSystem2579_SubSystem2581_SubSystem2593_Assignment_1"
  Inside_DSR/1 -> Assignment/1  "mdl4_SubSystem2493_SubSystem2577_SubSystem2579_SubSystem2581_SubSystem2593_Inside_DSR_1"
  input/1 -> Assignment/2
  element/1 -> Assignment/3

== system mdl4/SubSystem2493/SubSystem2577/SubSystem2579/SubSystem2581/SubSystem2594 ==
  note: ***編集禁止***
  input : Inport
  element : Inport  Port=2
  Assignment : Assignment  IndexOptions=Index vector (port)  OutputSizes=[1 1]
  Inside_DSR : DataStoreRead  DataStoreName=DSM281
  Inside_DSW : DataStoreWrite  DataStoreName=DSM281
  wires:
  Assignment/1 -> Inside_DSW/1  "mdl4_SubSystem2493_SubSystem2577_SubSystem2579_SubSystem2581_SubSystem2594_Assignment_1"
  Inside_DSR/1 -> Assignment/1  "mdl4_SubSystem2493_SubSystem2577_SubSystem2579_SubSystem2581_SubSystem2594_Inside_DSR_1"
  input/1 -> Assignment/2
  element/1 -> Assignment/3

== system mdl4/SubSystem2493/SubSystem2494/SubSystem2500/SubSystem2504/SubSystem2507/SubSystem2508 ==
  note: ***編集禁止***
  In1 : Inport
  In2 : Inport  Port=2
  RO1 : RelationalOperator  Operator===  InputSameDT=on
  single1 : DataTypeConversion  OutDataTypeStr=single  SaturateOnIntegerOverflow=on  RndMeth=Zero
  single2 : DataTypeConversion  OutDataTypeStr=single  SaturateOnIntegerOverflow=on  RndMeth=Zero
  Out1 : Outport
  wires:
  RO1/1 -> Out1/1  "mdl4_SubSystem2493_SubSystem2494_SubSystem2500_SubSystem2504_SubSystem2507_SubSystem2508_RO1_1"
  In2/1 -> single2/1
  In1/1 -> single1/1
  single1/1 -> RO1/1  "mdl4_SubSystem2493_SubSystem2494_SubSystem2500_SubSystem2504_SubSystem2507_SubSystem2508_single1_1"
  single2/1 -> RO1/2  "mdl4_SubSystem2493_SubSystem2494_SubSystem2500_SubSystem2504_SubSystem2507_SubSystem2508_single2_1"

== system mdl4/SubSystem2493/SubSystem2494/SubSystem2500/SubSystem2504/SubSystem2509/SubSystem2510 ==
  note: ***編集禁止***
  In1 : Inport
  In2 : Inport  Port=2
  RO1 : RelationalOperator  Operator===  InputSameDT=on
  single1 : DataTypeConversion  OutDataTypeStr=single  SaturateOnIntegerOverflow=on  RndMeth=Zero
  single2 : DataTypeConversion  OutDataTypeStr=single  SaturateOnIntegerOverflow=on  RndMeth=Zero
  Out1 : Outport
  wires:
  single2/1 -> RO1/2  "mdl4_SubSystem2493_SubSystem2494_SubSystem2500_SubSystem2504_SubSystem2509_SubSystem2510_single2_1"
  single1/1 -> RO1/1  "mdl4_SubSystem2493_SubSystem2494_SubSystem2500_SubSystem2504_SubSystem2509_SubSystem2510_single1_1"
  In1/1 -> single1/1
  In2/1 -> single2/1
  RO1/1 -> Out1/1  "mdl4_SubSystem2493_SubSystem2494_SubSystem2500_SubSystem2504_SubSystem2509_SubSystem2510_RO1_1"

== system mdl4/SubSystem2493/SubSystem2494/SubSystem2500/SubSystem2504/SubSystem2511/SubSystem2512 ==
  note: ***編集禁止***
  element : Inport
  Inside_DSR : DataStoreRead  DataStoreName=DSM258
  Selector : Selector  IndexOptions=Index vector (port)  Indices=[1 3]
  Output : Outport
  wires:
  Inside_DSR/1 -> Selector/1  "mdl4_SubSystem2493_SubSystem2494_SubSystem2500_SubSystem2504_SubSystem2511_SubSystem2512_Inside_DSR_1"
  element/1 -> Selector/2
  Selector/1 -> Output/1  "mdl4_SubSystem2493_SubSystem2494_SubSystem2500_SubSystem2504_SubSystem2511_SubSystem2512_Selector_1"

== system mdl4/SubSystem2493/SubSystem2494/SubSystem2500/SubSystem2504/SubSystem2511/SubSystem2513 ==
  note: ***編集禁止***
  element : Inport
  Inside_DSR : DataStoreRead  DataStoreName=DSM259
  Selector : Selector  IndexOptions=Index vector (port)  Indices=[1 3]
  Output : Outport
  wires:
  Selector/1 -> Output/1  "mdl4_SubSystem2493_SubSystem2494_SubSystem2500_SubSystem2504_SubSystem2511_SubSystem2513_Selector_1"
  element/1 -> Selector/2
  Inside_DSR/1 -> Selector/1  "mdl4_SubSystem2493_SubSystem2494_SubSystem2500_SubSystem2504_SubSystem2511_SubSystem2513_Inside_DSR_1"

== system mdl4/SubSystem2493/SubSystem2494/SubSystem2500/SubSystem2504/SubSystem2511/SubSystem2514 ==
  note: ***編集禁止***
  element : Inport
  Inside_DSR : DataStoreRead  DataStoreName=DSM300
  Selector : Selector  IndexOptions=Index vector (port)  Indices=[1 3]
  Output : Outport
  wires:
  Inside_DSR/1 -> Selector/1  "mdl4_SubSystem2493_SubSystem2494_SubSystem2500_SubSystem2504_SubSystem2511_SubSystem2514_Inside_DSR_1"
  element/1 -> Selector/2
  Selector/1 -> Output/1  "mdl4_SubSystem2493_SubSystem2494_SubSystem2500_SubSystem2504_SubSystem2511_SubSystem2514_Selector_1"

== system mdl4/SubSystem2493/SubSystem2494/SubSystem2500/SubSystem2504/SubSystem2511/SubSystem2515 ==
  note: ***編集禁止***
  input : Inport
  element : Inport  Port=2
  Assignment : Assignment  IndexOptions=Index vector (port)  OutputSizes=[1 1]
  Inside_DSR : DataStoreRead  DataStoreName=DSM302
  Inside_DSW : DataStoreWrite  DataStoreName=DSM302
  wires:
  element/1 -> Assignment/3
  input/1 -> Assignment/2
  Inside_DSR/1 -> Assignment/1  "mdl4_SubSystem2493_SubSystem2494_SubSystem2500_SubSystem2504_SubSystem2511_SubSystem2515_Inside_DSR_1"
  Assignment/1 -> Inside_DSW/1  "mdl4_SubSystem2493_SubSystem2494_SubSystem2500_SubSystem2504_SubSystem2511_SubSystem2515_Assignment_1"

== system mdl4/SubSystem2493/SubSystem2494/SubSystem2500/SubSystem2504/SubSystem2511/SubSystem2516 ==
  note: ***編集禁止***
  input : Inport
  element : Inport  Port=2
  Assignment : Assignment  IndexOptions=Index vector (port)  OutputSizes=[1 1]
  Inside_DSR : DataStoreRead  DataStoreName=DSM301
  Inside_DSW : DataStoreWrite  DataStoreName=DSM301
  wires:
  Assignment/1 -> Inside_DSW/1  "mdl4_SubSystem2493_SubSystem2494_SubSystem2500_SubSystem2504_SubSystem2511_SubSystem2516_Assignment_1"
  Inside_DSR/1 -> Assignment/1  "mdl4_SubSystem2493_SubSystem2494_SubSystem2500_SubSystem2504_SubSystem2511_SubSystem2516_Inside_DSR_1"
  input/1 -> Assignment/2
  element/1 -> Assignment/3

== system mdl4/SubSystem2493/SubSystem2494/SubSystem2500/SubSystem2504/SubSystem2511/SubSystem2517 ==
  note: ***編集禁止***
  input : Inport
  element : Inport  Port=2
  Assignment : Assignment  IndexOptions=Index vector (port)  OutputSizes=[1 1]
  Inside_DSR : DataStoreRead  DataStoreName=DSM303
  Inside_DSW : DataStoreWrite  DataStoreName=DSM303
  wires:
  Assignment/1 -> Inside_DSW/1  "mdl4_SubSystem2493_SubSystem2494_SubSystem2500_SubSystem2504_SubSystem2511_SubSystem2517_Assignment_1"
  Inside_DSR/1 -> Assignment/1  "mdl4_SubSystem2493_SubSystem2494_SubSystem2500_SubSystem2504_SubSystem2511_SubSystem2517_Inside_DSR_1"
  input/1 -> Assignment/2
  element/1 -> Assignment/3

== system mdl4/SubSystem2493/SubSystem2494/SubSystem2500/SubSystem2504/SubSystem2511/SubSystem2518 ==
  note: ***編集禁止***
  input : Inport
  element : Inport  Port=2
  Assignment : Assignment  IndexOptions=Index vector (port)  OutputSizes=[1 1]
  Inside_DSR : DataStoreRead  DataStoreName=DSM300
  Inside_DSW : DataStoreWrite  DataStoreName=DSM300
  wires:
  element/1 -> Assignment/3
  input/1 -> Assignment/2
  Inside_DSR/1 -> Assignment/1  "mdl4_SubSystem2493_SubSystem2494_SubSystem2500_SubSystem2504_SubSystem2511_SubSystem2518_Inside_DSR_1"
  Assignment/1 -> Inside_DSW/1  "mdl4_SubSystem2493_SubSystem2494_SubSystem2500_SubSystem2504_SubSystem2511_SubSystem2518_Assignment_1"

== system mdl4/SubSystem2493/SubSystem2494/SubSystem2500/SubSystem2504/SubSystem2519/SubSystem2520 ==
  note: ***編集禁止***
  element : Inport
  Inside_DSR : DataStoreRead  DataStoreName=DSM114
  Selector : Selector  IndexOptions=Index vector (port)  Indices=[1 3]
  Output : Outport
  wires:
  Inside_DSR/1 -> Selector/1  "mdl4_SubSystem2493_SubSystem2494_SubSystem2500_SubSystem2504_SubSystem2519_SubSystem2520_Inside_DSR_1"
  element/1 -> Selector/2
  Selector/1 -> Output/1  "mdl4_SubSystem2493_SubSystem2494_SubSystem2500_SubSystem2504_SubSystem2519_SubSystem2520_Selector_1"

== system mdl4/SubSystem2493/SubSystem2494/SubSystem2500/SubSystem2504/SubSystem2519/SubSystem2521 ==
  note: ***編集禁止***
  element : Inport
  Inside_DSR : DataStoreRead  DataStoreName=DSM105
  Selector : Selector  IndexOptions=Index vector (port)  Indices=[1 3]
  Output : Outport
  wires:
  Inside_DSR/1 -> Selector/1  "mdl4_SubSystem2493_SubSystem2494_SubSystem2500_SubSystem2504_SubSystem2519_SubSystem2521_Inside_DSR_1"
  element/1 -> Selector/2
  Selector/1 -> Output/1  "mdl4_SubSystem2493_SubSystem2494_SubSystem2500_SubSystem2504_SubSystem2519_SubSystem2521_Selector_1"

== system mdl4/SubSystem2493/SubSystem2494/SubSystem2500/SubSystem2504/SubSystem2519/SubSystem2522 ==
  note: ***編集禁止***
  element : Inport
  Inside_DSR : DataStoreRead  DataStoreName=DSM111
  Selector : Selector  IndexOptions=Index vector (port)  Indices=[1 3]
  Output : Outport
  wires:
  Inside_DSR/1 -> Selector/1  "mdl4_SubSystem2493_SubSystem2494_SubSystem2500_SubSystem2504_SubSystem2519_SubSystem2522_Inside_DSR_1"
  element/1 -> Selector/2
  Selector/1 -> Output/1  "mdl4_SubSystem2493_SubSystem2494_SubSystem2500_SubSystem2504_SubSystem2519_SubSystem2522_Selector_1"

== system mdl4/SubSystem2493/SubSystem2494/SubSystem2500/SubSystem2504/SubSystem2519/SubSystem2523 ==
  note: ***編集禁止***
  element : Inport
  Inside_DSR : DataStoreRead  DataStoreName=DSM113
  Selector : Selector  IndexOptions=Index vector (port)  Indices=[1 3]
  Output : Outport
  wires:
  Inside_DSR/1 -> Selector/1  "mdl4_SubSystem2493_SubSystem2494_SubSystem2500_SubSystem2504_SubSystem2519_SubSystem2523_Inside_DSR_1"
  element/1 -> Selector/2
  Selector/1 -> Output/1  "mdl4_SubSystem2493_SubSystem2494_SubSystem2500_SubSystem2504_SubSystem2519_SubSystem2523_Selector_1"

== system mdl4/SubSystem2493/SubSystem2494/SubSystem2500/SubSystem2504/SubSystem2519/SubSystem2524 ==
  note: ***編集禁止***
  element : Inport
  Inside_DSR : DataStoreRead  DataStoreName=DSM118
  Selector : Selector  IndexOptions=Index vector (port)  Indices=[1 3]
  Output : Outport
  wires:
  Inside_DSR/1 -> Selector/1  "mdl4_SubSystem2493_SubSystem2494_SubSystem2500_SubSystem2504_SubSystem2519_SubSystem2524_Inside_DSR_1"
  element/1 -> Selector/2
  Selector/1 -> Output/1  "mdl4_SubSystem2493_SubSystem2494_SubSystem2500_SubSystem2504_SubSystem2519_SubSystem2524_Selector_1"

== system mdl4/SubSystem2493/SubSystem2494/SubSystem2500/SubSystem2504/SubSystem2519/SubSystem2525 ==
  note: ***編集禁止***
  element : Inport
  Inside_DSR : DataStoreRead  DataStoreName=DSM117
  Selector : Selector  IndexOptions=Index vector (port)  Indices=[1 3]
  Output : Outport
  wires:
  Inside_DSR/1 -> Selector/1  "mdl4_SubSystem2493_SubSystem2494_SubSystem2500_SubSystem2504_SubSystem2519_SubSystem2525_Inside_DSR_1"
  element/1 -> Selector/2
  Selector/1 -> Output/1  "mdl4_SubSystem2493_SubSystem2494_SubSystem2500_SubSystem2504_SubSystem2519_SubSystem2525_Selector_1"

== system mdl4/SubSystem2493/SubSystem2494/SubSystem2500/SubSystem2504/SubSystem2519/SubSystem2526 ==
  note: ***編集禁止***
  element : Inport
  Inside_DSR : DataStoreRead  DataStoreName=DSM121
  Selector : Selector  IndexOptions=Index vector (port)  Indices=[1 3]
  Output : Outport
  wires:
  Inside_DSR/1 -> Selector/1  "mdl4_SubSystem2493_SubSystem2494_SubSystem2500_SubSystem2504_SubSystem2519_SubSystem2526_Inside_DSR_1"
  element/1 -> Selector/2
  Selector/1 -> Output/1  "mdl4_SubSystem2493_SubSystem2494_SubSystem2500_SubSystem2504_SubSystem2519_SubSystem2526_Selector_1"

== system mdl4/SubSystem2493/SubSystem2494/SubSystem2500/SubSystem2504/SubSystem2519/SubSystem2527 ==
  note: ***編集禁止***
  element : Inport
  Inside_DSR : DataStoreRead  DataStoreName=DSM124
  Selector : Selector  IndexOptions=Index vector (port)  Indices=[1 3]
  Output : Outport
  wires:
  Inside_DSR/1 -> Selector/1  "mdl4_SubSystem2493_SubSystem2494_SubSystem2500_SubSystem2504_SubSystem2519_SubSystem2527_Inside_DSR_1"
  element/1 -> Selector/2
  Selector/1 -> Output/1  "mdl4_SubSystem2493_SubSystem2494_SubSystem2500_SubSystem2504_SubSystem2519_SubSystem2527_Selector_1"
